simulink model "bpsk_sim"  (R2018b)
settings: Solver=VariableStepAuto  StartTime=0.0  StopTime=0  RelTol=1e-3
values from neighbouring files (symbols this model uses):
  snr = SNR_dB(i)    [simout_bpsk.m]
libraries: commrandsrc3 x1
settings Model: Creator=DSP_08  LastModifiedBy=DSP_08

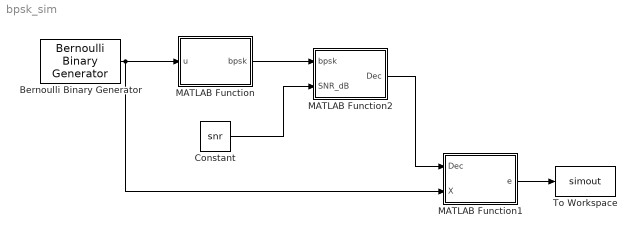
== system bpsk_sim ==
  Bernoulli Binary Generator : commrandsrc3/Bernoulli Binary Generator  ProbabilityOfZero=0.5  SeedSource=Auto  Seed=0  SampleTime=1  SamplesPerFrame=100000  OutputDataType=double  SimulateUsing=Interpreted execution
  Constant : Constant  Value=snr
  MATLAB Function : MATLAB Function  TreatAsAtomicUnit=on
  MATLAB Function1 : MATLAB Function  TreatAsAtomicUnit=on
  MATLAB Function2 : MATLAB Function  TreatAsAtomicUnit=on
  To Workspace : ToWorkspace  VariableName=simout  SampleTime=-1
      settings: Save2DSignal=2-D array (concatenate along first dimension)
  wires:
  Constant/1 -> MATLAB Function2/2(SNR_dB)
  MATLAB Function/1(bpsk) -> MATLAB Function2/1(bpsk)
  MATLAB Function2/1(Dec) -> MATLAB Function1/1(Dec)
  MATLAB Function1/1(e) -> To Workspace/1
  Bernoulli Binary Generator/1 -> MATLAB Function1/2(X), MATLAB Function/1(u)

== matlab function bpsk_sim/MATLAB Function1 ==
  data: Dec input; e output; X input
function e = fcn(Dec,X)

    N = length(Dec);
    X_rcvd = zeros(1,N);
    X = transpose(X);
    for j = 1:N
        if Dec(j) > 0
            X_rcvd(j) = 1;
        else
            X_rcvd(j) = 0;
        end
    end
    e = sum(abs(X-X_rcvd))/N;
    
end

== matlab function bpsk_sim/MATLAB Function ==
  data: u input; bpsk output
function bpsk = fcn(u)

    X = transpose(u);
    N = length(u);
    bpsk = zeros(1,N);
    for i = 1:N
        if X(i) == 0
            bpsk(i) = -1;
        else
            bpsk(i) = 1;
        end
    end

end

== matlab function bpsk_sim/MATLAB Function2 ==
  data: bpsk input; Dec output; SNR_dB input
function Dec = fcn(bpsk,SNR_dB)

N = length(bpsk);
y1 = complex(randn(1,N),randn(1,N));
y2 = complex(randn(1,N),randn(1,N));
Dec = complex(randn(1,N),randn(1,N));

    h1 = (1/sqrt(2)).*complex(randn(1,N),randn(1,N));
    h2 = (1/sqrt(2)).*complex(randn(1,N),randn(1,N));
    n1 = complex(randn(1,N),randn(1,N));
    n2 = complex(randn(1,N),randn(1,N));
    normsq_h = h1.*conj(h1) + h2.*conj(h2);
    SNR_lin = 10^(SNR_dB/10);
    sigma = 1/sqrt(SNR_lin);
    y1 = h1.*bpsk + sigma*n1;
    y2 = h2.*bpsk + sigma*n2;
    Dec = ((conj(h1).*y1)+(conj(h2).*y2))./normsq_h;

end
